simulink model "lqs2a1"  (R2022b)
settings: Solver=FixedStepAuto  StartTime=0.0  StopTime=20  FixedStep=0.05  RelTol=1e-3
model workspace (MAT data in the model file):
  Q = Simulink.Parameter
  Q.Value = [2 1]
  Q.DataType = 'auto'
  Q.Complexity = 'real'
  Q.Dimensions = [1 2]
  R = Simulink.Parameter
  R.Value = 1
  R.DataType = 'auto'
  R.Complexity = 'real'
  R.Dimensions = [1 1]
  a_max = 5
  a_min = -5
  adva_max = 0.001
  adva_min = -0.001
  x_ini = Simulink.Parameter
  x_ini.Value = [0.05 0.05]
  x_ini.DataType = 'auto'
  x_ini.Complexity = 'real'
  x_ini.Dimensions = [1 2]
libraries: simulink x1
settings Model: TunableVars=a_max,a_min,adva_max,adva_min,x_ini,x_max,x_min  TunableVarsStorageClass=Auto,Auto,Auto,Auto,Auto,Auto,Auto  TunableVarsTypeQualifier=,,,,,,  ParameterArgumentNames=Q,R,x_ini  Creator=hjzsj  LastModifiedBy=Genjin Xie
settings ConfigSet: Description=Config for code generation python binding.
settings SolverCC: AlgebraicLoopSolver=TrustRegion
settings OptimizationCC: DefaultParameterBehavior=Inlined  UseDivisionForNetSlopeComputation=on  UseFloatMulNetSlope=on  StrengthReduction=on  PassReuseOutputArgsAs=Individual arguments  ZeroExternalMemoryAtStartup=off  ZeroInternalMemoryAtStartup=off  NoFixptDivByZeroProtection=on  EfficientFloat2IntCast=on  OptimizeBlockOrder=speed  OptimizationPriority=Speed  OptimizationCustomize=off  MultiThreadedLoops=on  EfficientTunableParamExpr=on
settings DebuggingCC: ParameterTunabilityLossMsg=error  UnconnectedInputMsg=warning  UnconnectedOutputMsg=warning  UnconnectedLineMsg=warning  SFMachineParentedDataDiag=warning  ArithmeticOperatorsInVariantConditions=warning
settings HardwareCC: ProdLongLongMode=on  TargetPreprocMaxBitsSint=64  TargetPreprocMaxBitsUint=64
settings ModelReferenceCC: EnableRefExpFcnMdlSchedulingChecks=on
settings SFSimCC: MATLABDynamicMemAlloc=off  CustomCodeUndefinedFunction=UseInterfaceOnly  SimTargetLang=C++
settings RTWCC: Description=Embedded Coder  SystemTargetFile=ert.tlc  GenCodeOnly=on  TemplateMakefile=ert_default_tmf  PostCodeGenCommand=slxpy.postprocess(modelName,buildInfo)  RetainRTWFile=on  PortableWordSizes=on  TargetLang=C++
settings CodeAppCC: ForceParamTrailComments=on  CommentStyle=Multi-line  IgnoreCustomStorageClasses=off  MaxIdLength=64  OperatorAnnotations=on  SimulinkDataObjDesc=on  SFDataObjDesc=on  MATLABFcnDesc=on  MangleLength=4  InsertBlockDesc=on  StateflowObjectComments=on  MATLABSourceComments=on
settings ERTTargetCC: TargetLangStandard=C++11 (ISO)  SupportAbsoluteTime=off  CodeInterfacePackaging=C++ class  SupportNonFinite=off  SupportComplex=off  SupportContinuousTime=on  InlinedParameterPlacement=NonHierarchical  RootIOFormat=Structure reference  ERTCustomFileTemplate=example_file_process.tlc

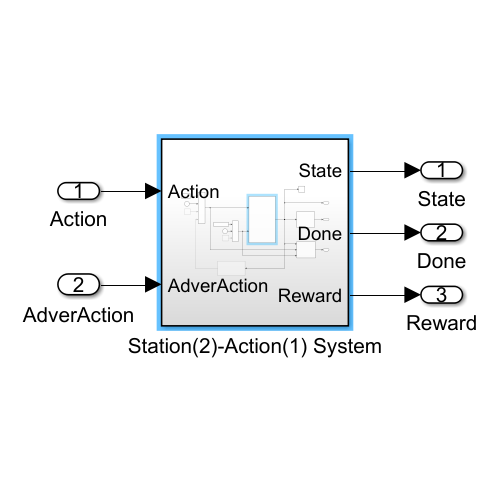
[thumbnail: Simulink's stored preview of the top-level diagram]
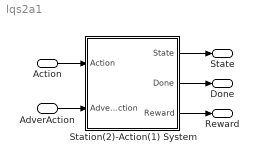
== system lqs2a1 ==
  Action : Inport
  AdverAction : Inport  Port=2
  Station(2)-Action(1) System : Subsystem
  State : Outport
  Done : Outport  Port=2
  Reward : Outport  Port=3
  wires:
  Station(2)-Action(1) System/1(State) -> State/1
  Station(2)-Action(1) System/2(Done) -> Done/1
  Action/1 -> Station(2)-Action(1) System/1(Action)
  Station(2)-Action(1) System/3(Reward) -> Reward/1
  AdverAction/1 -> Station(2)-Action(1) System/2(AdverAction)

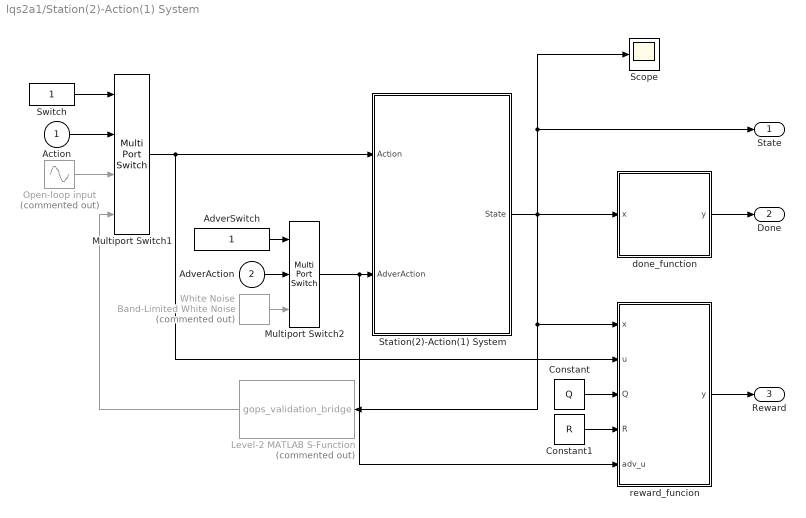
== system lqs2a1/Station(2)-Action(1) System ==
  Action : Inport
  AdverAction : Inport  Port=2
  AdverSwitch : Constant
  Constant : Constant  Value=Q
  Constant1 : Constant  Value=R
  Level-2 MATLAB S-Function : M-S-Function  Commented=on  FunctionName=gops_validation_bridge  Parameters="\"C:\\Users\\Genjin Xie\\Desktop\\14dofModel\\model-2021b\\NN_controller_MLP.pt\""
  Multiport Switch1 : MultiPortSwitch  SaturateOnIntegerOverflow=off  InputSameDT=off
  Multiport Switch2 : MultiPortSwitch  Inputs=2  SaturateOnIntegerOverflow=off  InputSameDT=off
  Open-loop input : Sin  Commented=on  SampleTime=0
  Scope : Scope
  Station(2)-Action(1) System : Subsystem
  Switch : Constant
  White Noise : simulink/Sources/Band-Limited White Noise  Commented=on  Cov=[0.5]  Ts=0.02  seed=[23341]
  done_function : MATLAB Function  TreatAsAtomicUnit=on
  reward_funcion : MATLAB Function  TreatAsAtomicUnit=on
  State : Outport
  Done : Outport  Port=2
  Reward : Outport  Port=3
  wires:
  done_function/1(y) -> Done/1
  reward_funcion/1(y) -> Reward/1
  Level-2 MATLAB S-Function/1 -> Multiport Switch1/4
  Switch/1 -> Multiport Switch1/1
  Action/1 -> Multiport Switch1/2
  Station(2)-Action(1) System/1(State) -> done_function/1(x), State/1, Scope/1, Level-2 MATLAB S-Function/1, reward_funcion/1(x)
  Multiport Switch1/1 -> reward_funcion/2(u), Station(2)-Action(1) System/1(Action)
  Open-loop input/1 -> Multiport Switch1/3
  Multiport Switch2/1 -> reward_funcion/5(adv_u), Station(2)-Action(1) System/2(AdverAction)
  AdverSwitch/1 -> Multiport Switch2/1
  White Noise/1 -> Multiport Switch2/3
  AdverAction/1 -> Multiport Switch2/2
  Constant/1 -> reward_funcion/3(Q)
  Constant1/1 -> reward_funcion/4(R)

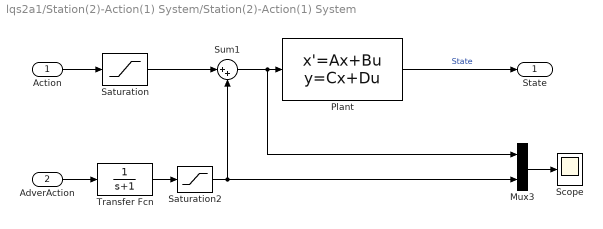
== system lqs2a1/Station(2)-Action(1) System/Station(2)-Action(1) System ==
  Action : Inport
  AdverAction : Inport  Port=2
  Mux3 : Mux  Inputs=2
  Plant : StateSpace  A=[0 1 ;0 0]  B=[0; 1]  C=[1 0;0 1]  D=zeros(2,1)  InitialCondition=x_ini
  Saturation : Saturate  UpperLimit=a_max  LowerLimit=a_min
  Saturation2 : Saturate  UpperLimit=adva_max  LowerLimit=adva_min
  Scope : Scope
  Sum1 : Sum  Inputs=|++
  Transfer Fcn : TransferFcn  Denominator=[1 1]
  State : Outport
  wires:
  Action/1 -> Saturation/1
  Transfer Fcn/1 -> Saturation2/1
  Mux3/1 -> Scope/1
  AdverAction/1 -> Transfer Fcn/1
  Saturation2/1 -> Sum1/2, Mux3/2
  Plant/1 -> State/1  "State"
  Saturation/1 -> Sum1/1
  Sum1/1 -> Mux3/1, Plant/1

== matlab function lqs2a1/Station(2)-Action(1) System/done_function ==
  data: x input; y output
function y = fcn(x)
done = (  (abs(x(1))>20) || ((abs(x(1)-0)<-20) && (abs(x(2))<-20)) || (abs(x(2))>20) );
y = done;

== matlab function lqs2a1/Station(2)-Action(1) System/reward_funcion ==
  data: x input; y output; u input; Q input; R input; adv_u input
function y = fcn(x, u, Q, R, adv_u)
reward = -Q(1)*(x(1)-0)^2-Q(2)*(x(2)-0)^2-R*u^2;
y = reward;
